simulink model "EEE_Lab2_CSE21180"  (R2024b)
settings: Solver=VariableStepAuto  StartTime=0.0  StopTime=10.0  RelTol=1e-3
libraries: spsCurrentMeasurementLib x9, spsSeriesRLCBranchLib x9, spsDCVoltageSourceLib x4, sps_lib x1
settings Model: Creator=surmy  LastModifiedBy=surmy

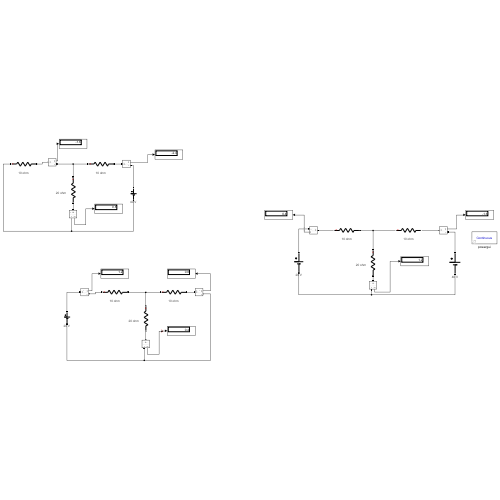
[thumbnail: Simulink's stored preview of the top-level diagram]
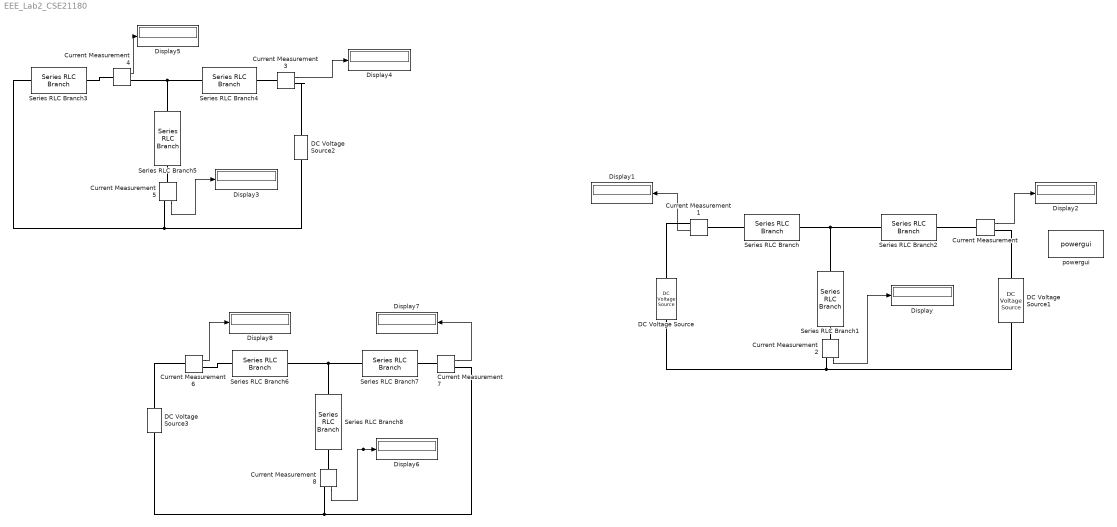
== system EEE_Lab2_CSE21180 ==
  Current Measurement{,1..8} (9 alike) : spsCurrentMeasurementLib/Current Measurement  PhasorSimulation=off  OutputType=Complex  PSBequivalent=0
  DC Voltage Source : spsDCVoltageSourceLib/DC Voltage Source  Amplitude=20  Measurements=None
      settings: AttributesFormatString=20 V
  DC Voltage Source1 : spsDCVoltageSourceLib/DC Voltage Source  Amplitude=40  Measurements=None
      settings: AttributesFormatString=40 V
  DC Voltage Source2 : spsDCVoltageSourceLib/DC Voltage Source  Amplitude=40  Measurements=None
      settings: AttributesFormatString=40 V
  DC Voltage Source3 : spsDCVoltageSourceLib/DC Voltage Source  Amplitude=20  Measurements=None
      settings: AttributesFormatString=20 V
  Display{,1..8} (9 alike) : Display
  Series RLC Branch{,2..4,6..7} (6 alike) : spsSeriesRLCBranchLib/Series RLC Branch  LConnTagsString=__new0  RConnTagsString=__new0  BranchType=R  Resistance=10  Inductance=1e-3  SetiL0=off  InitialCurrent=0  Capacitance=1e-6  Setx0=off  InitialVoltage=0  Measurements=None
      settings: AttributesFormatString=10 ohm
  Series RLC Branch1 : spsSeriesRLCBranchLib/Series RLC Branch  LConnTagsString=__new0  RConnTagsString=__new0  BranchType=R  Resistance=20  Inductance=1e-3  SetiL0=off  InitialCurrent=0  Capacitance=1e-6  Setx0=off  InitialVoltage=0  Measurements=None
      settings: AttributesFormatString=20 ohm
  Series RLC Branch5 : spsSeriesRLCBranchLib/Series RLC Branch  LConnTagsString=__new0  RConnTagsString=__new0  BranchType=R  Resistance=20  Inductance=1e-3  SetiL0=off  InitialCurrent=0  Capacitance=1e-6  Setx0=off  InitialVoltage=0  Measurements=None
      settings: AttributesFormatString=20 ohm
  Series RLC Branch8 : spsSeriesRLCBranchLib/Series RLC Branch  LConnTagsString=__new0  RConnTagsString=__new0  BranchType=R  Resistance=20  Inductance=1e-3  SetiL0=off  InitialCurrent=0  Capacitance=1e-6  Setx0=off  InitialVoltage=0  Measurements=None
      settings: AttributesFormatString=20 ohm
  powergui : sps_lib/powergui  Priority=1  SimulationMode=Continuous  SampleTime=50e-6  frequency=60  Iterations=50  frequencyindice=0  Pbase=100e6  ErrMax=1e-4  UnitsV=kV  UnitsW=MW  buscounter=0  FunctionMessages=off  echomessages=off  EnableUseOfTLC=off  CurrentSourceSwitches=off  DisableSnubberDevices=off  DisableRonSwitches=off  DisableVfSwitches=off  DisplayEquations=off  AutomaticDiscreteSolvers=off  SolverType=Tustin/Backward Euler (TBE)  Interpol=off  ExternalGateDelay=off  methode=off  Ts=100  x0status=blocks  SPID=on  SwTol=0  HookPort=off  NonlinearTolerance=1e-4  nMaxIteration=100  ContinueOnMaxIteration=off  RestoreLinks=warning  ResistiveCurrentMeasurement=off  Frange=[0:2:500]  Ylog=off  Xlog=on  ShowGrid=off  save=off  variable=ZData  structure=0  ZoomFFT=off  StartTime=0.0  cycles=1  DisplayStyle=1  fundamental=60  FreqAxis=off  MaxFrequency=1000  frequencyindicesteady=1  RmsSteady=1  display=off
  wires:
  Current Measurement2/1 -> Display/1
  Current Measurement/1 -> Display2/1
  Current Measurement5/1 -> Display3/1
  Current Measurement3/1 -> Display4/1
  Current Measurement4/1 -> Display5/1
  Current Measurement8/1 -> Display6/1
  Current Measurement6/1 -> Display8/1
  Current Measurement7/1 -> Display7/1
  Current Measurement1/1 -> Display1/1
  connections:
  Series RLC Branch1/LConn1 -- Series RLC Branch2/LConn1 -- Series RLC Branch/RConn1
  DC Voltage Source/LConn1 -- Current Measurement2/RConn1 -- DC Voltage Source1/LConn1
  Current Measurement2/LConn1 -- Series RLC Branch1/RConn1
  Current Measurement/LConn1 -- Series RLC Branch2/RConn1
  Current Measurement/RConn1 -- DC Voltage Source1/RConn1
  DC Voltage Source2/LConn1 -- Current Measurement5/RConn1 -- Series RLC Branch3/LConn1
  Series RLC Branch5/LConn1 -- Series RLC Branch4/LConn1 -- Current Measurement4/RConn1
  Current Measurement7/RConn1 -- Current Measurement8/RConn1 -- DC Voltage Source3/LConn1
  Series RLC Branch6/RConn1 -- Series RLC Branch8/LConn1 -- Series RLC Branch7/LConn1
  Current Measurement5/LConn1 -- Series RLC Branch5/RConn1
  Current Measurement3/LConn1 -- Series RLC Branch4/RConn1
  Current Measurement3/RConn1 -- DC Voltage Source2/RConn1
  Current Measurement4/LConn1 -- Series RLC Branch3/RConn1
  Current Measurement6/RConn1 -- Series RLC Branch6/LConn1
  Current Measurement6/LConn1 -- DC Voltage Source3/RConn1
  Current Measurement7/LConn1 -- Series RLC Branch7/RConn1
  Current Measurement8/LConn1 -- Series RLC Branch8/RConn1
  Current Measurement1/LConn1 -- Series RLC Branch/LConn1
  Current Measurement1/RConn1 -- DC Voltage Source/RConn1
